simulink model "bacteriaPopulationStateflow"  (R2017b)
settings: Solver=FixedStepDiscrete  StartTime=0.0  StopTime=10.0  FixedStep=1  RelTol=1e-3
model workspace (MAT data in the model file):
  ContractValidatorBlocksMap = containers.Map
  ContractValidatorBlocksMap.serialization.keys = {'bacteriaPopulationStateflow/bacteriaPopulationSpec/validator', 'bacteriaPopulationStateflow1/bacteriaPopulationSpec/validator'}
  ContractValidatorBlocksMap.serialization.values{1}.block = 'bacteriaPopulationStateflow/bacteriaPopulationSpec/validator'
  ContractValidatorBlocksMap.serialization.values{1}.assumePorts = 1
  ContractValidatorBlocksMap.serialization.values{1}.guaranteePorts = 4
  ContractValidatorBlocksMap.serialization.values{1}.modeBlocksPorts = 3
  ContractValidatorBlocksMap.serialization.values{1}.portHandles.Inport = [309.000366211 310.00012207 311.00012207 312.00012207 313.00012207 314.00012207 315.00012207 316.00012207]
  ContractValidatorBlocksMap.serialization.values{1}.portHandles.Outport = 317.00012207
  ContractValidatorBlocksMap.serialization.values{1}.portHandles.Enable = []
  ContractValidatorBlocksMap.serialization.values{1}.portHandles.Trigger = []
  ContractValidatorBlocksMap.serialization.values{1}.portHandles.State = []
  ContractValidatorBlocksMap.serialization.values{1}.portHandles.LConn = []
  ContractValidatorBlocksMap.serialization.values{1}.portHandles.RConn = []
  ContractValidatorBlocksMap.serialization.values{1}.portHandles.Ifaction = []
  ContractValidatorBlocksMap.serialization.values{1}.portHandles.Reset = []
  ContractValidatorBlocksMap.serialization.values{1}.portConnectivity(1).Type = '1'
  ContractValidatorBlocksMap.serialization.values{1}.portConnectivity(1).Position = [360 -280]
  ContractValidatorBlocksMap.serialization.values{1}.portConnectivity(1).SrcBlock = 21.0001220703
  ContractValidatorBlocksMap.serialization.values{1}.portConnectivity(1).SrcPort = 0
  ContractValidatorBlocksMap.serialization.values{1}.portConnectivity(1).DstBlock = []
  ContractValidatorBlocksMap.serialization.values{1}.portConnectivity(1).DstPort = []
  ContractValidatorBlocksMap.serialization.values{1}.portConnectivity(2).Type = '2'
  ContractValidatorBlocksMap.serialization.values{1}.portConnectivity(2).Position = [360 -170]
  ContractValidatorBlocksMap.serialization.values{1}.portConnectivity(2).SrcBlock = 81.0001220703
  ContractValidatorBlocksMap.serialization.values{1}.portConnectivity(2).SrcPort = 0
  ContractValidatorBlocksMap.serialization.values{1}.portConnectivity(2).DstBlock = []
  ContractValidatorBlocksMap.serialization.values{1}.portConnectivity(2).DstPort = []
  ContractValidatorBlocksMap.serialization.values{1}.portConnectivity(3).Type = '3'
  ContractValidatorBlocksMap.serialization.values{1}.portConnectivity(3).Position = [360 -60]
  ContractValidatorBlocksMap.serialization.values{1}.portConnectivity(3).SrcBlock = 87.0003662109
  ContractValidatorBlocksMap.serialization.values{1}.portConnectivity(3).SrcPort = 0
  ContractValidatorBlocksMap.serialization.values{1}.portConnectivity(3).DstBlock = []
  ContractValidatorBlocksMap.serialization.values{1}.portConnectivity(3).DstPort = []
  ContractValidatorBlocksMap.serialization.values{1}.portConnectivity(4).Type = '4'
  ContractValidatorBlocksMap.serialization.values{1}.portConnectivity(4).Position = [360 50]
  ContractValidatorBlocksMap.serialization.values{1}.portConnectivity(4).SrcBlock = 99.0003662109
  ContractValidatorBlocksMap.serialization.values{1}.portConnectivity(4).SrcPort = 0
  ContractValidatorBlocksMap.serialization.values{1}.portConnectivity(4).DstBlock = []
  ContractValidatorBlocksMap.serialization.values{1}.portConnectivity(4).DstPort = []
  ContractValidatorBlocksMap.serialization.values{1}.portConnectivity(5).Type = '5'
  ContractValidatorBlocksMap.serialization.values{1}.portConnectivity(5).Position = [360 160]
  ContractValidatorBlocksMap.serialization.values{1}.portConnectivity(5).SrcBlock = 148.000366211
  ContractValidatorBlocksMap.serialization.values{1}.portConnectivity(5).SrcPort = 0
  ContractValidatorBlocksMap.serialization.values{1}.portConnectivity(5).DstBlock = []
  ContractValidatorBlocksMap.serialization.values{1}.portConnectivity(5).DstPort = []
  ContractValidatorBlocksMap.serialization.values{1}.portConnectivity(6).Type = '6'
  ContractValidatorBlocksMap.serialization.values{1}.portConnectivity(6).Position = [360 270]
  ContractValidatorBlocksMap.serialization.values{1}.portConnectivity(6).SrcBlock = 197.000366211
  ContractValidatorBlocksMap.serialization.values{1}.portConnectivity(6).SrcPort = 0
  ContractValidatorBlocksMap.serialization.values{1}.portConnectivity(6).DstBlock = []
  ContractValidatorBlocksMap.serialization.values{1}.portConnectivity(6).DstPort = []
  ContractValidatorBlocksMap.serialization.values{1}.portConnectivity(7).Type = '7'
  ContractValidatorBlocksMap.serialization.values{1}.portConnectivity(7).Position = [360 380]
  ContractValidatorBlocksMap.serialization.values{1}.portConnectivity(7).SrcBlock = 27.0003662109
  ContractValidatorBlocksMap.serialization.values{1}.portConnectivity(7).SrcPort = 0
  ContractValidatorBlocksMap.serialization.values{1}.portConnectivity(7).DstBlock = []
  ContractValidatorBlocksMap.serialization.values{1}.portConnectivity(7).DstPort = []
  ContractValidatorBlocksMap.serialization.values{1}.portConnectivity(8).Type = '8'
  ContractValidatorBlocksMap.serialization.values{1}.portConnectivity(8).Position = [360 490]
  ContractValidatorBlocksMap.serialization.values{1}.portConnectivity(8).SrcBlock = 238.000366211
  ContractValidatorBlocksMap.serialization.values{1}.portConnectivity(8).SrcPort = 0
  ContractValidatorBlocksMap.serialization.values{1}.portConnectivity(8).DstBlock = []
  ContractValidatorBlocksMap.serialization.values{1}.portConnectivity(8).DstPort = []
  ContractValidatorBlocksMap.serialization.values{1}.portConnectivity(9).Type = '1'
  ContractValidatorBlocksMap.serialization.values{1}.portConnectivity(9).Position = [500 105]
  ContractValidatorBlocksMap.serialization.values{1}.portConnectivity(9).SrcBlock = []
  ContractValidatorBlocksMap.serialization.values{1}.portConnectivity(9).SrcPort = []
  ContractValidatorBlocksMap.serialization.values{1}.portConnectivity(9).DstBlock = [250.00012207 20.0001220703]
  ContractValidatorBlocksMap.serialization.values{1}.portConnectivity(9).DstPort = [0 0]
  ContractValidatorBlocksMap.serialization.values{2}.block = 'bacteriaPopulationStateflow1/bacteriaPopulationSpec/validator'
  ContractValidatorBlocksMap.serialization.values{2}.assumePorts = 1
  ContractValidatorBlocksMap.serialization.values{2}.guaranteePorts = 4
  ContractValidatorBlocksMap.serialization.values{2}.modeBlocksPorts = 3
  ContractValidatorBlocksMap.serialization.values{2}.portHandles.Inport = [309.001586914 310.001220703 311.000854492 312.000976562 313.000976562 314.001098633 315.000976562 316.000854492]
  ContractValidatorBlocksMap.serialization.values{2}.portHandles.Outport = 317.001098633
  ContractValidatorBlocksMap.serialization.values{2}.portHandles.Enable = []
  ContractValidatorBlocksMap.serialization.values{2}.portHandles.Trigger = []
  ContractValidatorBlocksMap.serialization.values{2}.portHandles.State = []
  ContractValidatorBlocksMap.serialization.values{2}.portHandles.LConn = []
  ContractValidatorBlocksMap.serialization.values{2}.portHandles.RConn = []
  ContractValidatorBlocksMap.serialization.values{2}.portHandles.Ifaction = []
  ContractValidatorBlocksMap.serialization.values{2}.portHandles.Reset = []
  ContractValidatorBlocksMap.serialization.values{2}.portConnectivity(1).Type = '1'
  ContractValidatorBlocksMap.serialization.values{2}.portConnectivity(1).Position = [360 -280]
  ContractValidatorBlocksMap.serialization.values{2}.portConnectivity(1).SrcBlock = 21.0007324219
  ContractValidatorBlocksMap.serialization.values{2}.portConnectivity(1).SrcPort = 0
  ContractValidatorBlocksMap.serialization.values{2}.portConnectivity(1).DstBlock = []
  ContractValidatorBlocksMap.serialization.values{2}.portConnectivity(1).DstPort = []
  ContractValidatorBlocksMap.serialization.values{2}.portConnectivity(2).Type = '2'
  ContractValidatorBlocksMap.serialization.values{2}.portConnectivity(2).Position = [360 -170]
  ContractValidatorBlocksMap.serialization.values{2}.portConnectivity(2).SrcBlock = 81.0010986328
  ContractValidatorBlocksMap.serialization.values{2}.portConnectivity(2).SrcPort = 0
  ContractValidatorBlocksMap.serialization.values{2}.portConnectivity(2).DstBlock = []
  ContractValidatorBlocksMap.serialization.values{2}.portConnectivity(2).DstPort = []
  ContractValidatorBlocksMap.serialization.values{2}.portConnectivity(3).Type = '3'
  ContractValidatorBlocksMap.serialization.values{2}.portConnectivity(3).Position = [360 -60]
  ContractValidatorBlocksMap.serialization.values{2}.portConnectivity(3).SrcBlock = 87.0009765625
  ContractValidatorBlocksMap.serialization.values{2}.portConnectivity(3).SrcPort = 0
  ContractValidatorBlocksMap.serialization.values{2}.portConnectivity(3).DstBlock = []
  ContractValidatorBlocksMap.serialization.values{2}.portConnectivity(3).DstPort = []
  ContractValidatorBlocksMap.serialization.values{2}.portConnectivity(4).Type = '4'
  ContractValidatorBlocksMap.serialization.values{2}.portConnectivity(4).Position = [360 50]
  ContractValidatorBlocksMap.serialization.values{2}.portConnectivity(4).SrcBlock = 99.0009765625
  ContractValidatorBlocksMap.serialization.values{2}.portConnectivity(4).SrcPort = 0
  ContractValidatorBlocksMap.serialization.values{2}.portConnectivity(4).DstBlock = []
  ContractValidatorBlocksMap.serialization.values{2}.portConnectivity(4).DstPort = []
  ContractValidatorBlocksMap.serialization.values{2}.portConnectivity(5).Type = '5'
  ContractValidatorBlocksMap.serialization.values{2}.portConnectivity(5).Position = [360 160]
  ContractValidatorBlocksMap.serialization.values{2}.portConnectivity(5).SrcBlock = 148.000976562
  ContractValidatorBlocksMap.serialization.values{2}.portConnectivity(5).SrcPort = 0
  ContractValidatorBlocksMap.serialization.values{2}.portConnectivity(5).DstBlock = []
  ContractValidatorBlocksMap.serialization.values{2}.portConnectivity(5).DstPort = []
  ContractValidatorBlocksMap.serialization.values{2}.portConnectivity(6).Type = '6'
  ContractValidatorBlocksMap.serialization.values{2}.portConnectivity(6).Position = [360 270]
  ContractValidatorBlocksMap.serialization.values{2}.portConnectivity(6).SrcBlock = 197.000976562
  ContractValidatorBlocksMap.serialization.values{2}.portConnectivity(6).SrcPort = 0
  ContractValidatorBlocksMap.serialization.values{2}.portConnectivity(6).DstBlock = []
  ContractValidatorBlocksMap.serialization.values{2}.portConnectivity(6).DstPort = []
  ContractValidatorBlocksMap.serialization.values{2}.portConnectivity(7).Type = '7'
  ContractValidatorBlocksMap.serialization.values{2}.portConnectivity(7).Position = [360 380]
  ContractValidatorBlocksMap.serialization.values{2}.portConnectivity(7).SrcBlock = 27.0018310547
  ContractValidatorBlocksMap.serialization.values{2}.portConnectivity(7).SrcPort = 0
  ContractValidatorBlocksMap.serialization.values{2}.portConnectivity(7).DstBlock = []
  ContractValidatorBlocksMap.serialization.values{2}.portConnectivity(7).DstPort = []
  ContractValidatorBlocksMap.serialization.values{2}.portConnectivity(8).Type = '8'
  ContractValidatorBlocksMap.serialization.values{2}.portConnectivity(8).Position = [360 490]
  ContractValidatorBlocksMap.serialization.values{2}.portConnectivity(8).SrcBlock = 238.000976562
  ContractValidatorBlocksMap.serialization.values{2}.portConnectivity(8).SrcPort = 0
  ContractValidatorBlocksMap.serialization.values{2}.portConnectivity(8).DstBlock = []
  ContractValidatorBlocksMap.serialization.values{2}.portConnectivity(8).DstPort = []
  ContractValidatorBlocksMap.serialization.values{2}.portConnectivity(9).Type = '1'
  ContractValidatorBlocksMap.serialization.values{2}.portConnectivity(9).Position = [500 105]
  ContractValidatorBlocksMap.serialization.values{2}.portConnectivity(9).SrcBlock = []
  ContractValidatorBlocksMap.serialization.values{2}.portConnectivity(9).SrcPort = []
  ContractValidatorBlocksMap.serialization.values{2}.portConnectivity(9).DstBlock = [250.000488281 20.0009765625]
  ContractValidatorBlocksMap.serialization.values{2}.portConnectivity(9).DstPort = [0 0]
  ContractValidatorBlocksMap.serialization.uniformity = 0
  ContractValidatorBlocksMap.serialization.keyType = 'char'
  ContractValidatorBlocksMap.serialization.valueType = 'any'
undefined symbols (not defined in the file or in its folder): contractAfterSimulation, ContractAssumeBlock, contractBeforeSimulation, ContractBlock, ContractEnsureBlock, ContractGuaranteeBlock, ContractModeBlock, ContractRequireBlock, ContractValidatorBlock, saveValidatorParameters
libraries: Kind x14, simulink x2
settings Model: Creator=Mudathir  LastModifiedBy=mudat
settings CodeAppCC: StateflowObjectComments=on

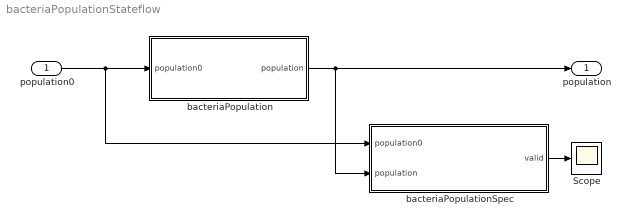
== system bacteriaPopulationStateflow ==
  population0 : Inport
  Scope : Scope
  bacteriaPopulation : Stateflow chart  TreatAsAtomicUnit=on
  bacteriaPopulationSpec : Subsystem  mask{ContractBlockType=ContractBlock}
      mask init:
      | set_param(gcb, 'LinkStatus', 'none');
      mask DialogControl DescTextVar Prompt: Contract block
      mask Display:
      | text(0.5, 0.5, '{\bf\fontsize{20}Contract}', 'hor', 'center', 'texmode','on');
      | blocks = find_system(gcb, 'LookUnderMasks','all', 'SearchDepth',1,'BlockType','Inport');
      | for i = 1 : length(blocks)
      |     blockName = get_param(blocks(i), 'Name');
      |     [path, blockName] = fileparts(char(blockName));
      |     port_label('input', i, blockName);
      | end
      | 
      | blocks = find_system(gcb, 'LookUnderMasks','all', 'SearchDepth',1,'BlockType','Outport');
      | for i = 1 : length(blocks)
      |     blockName = get_param(blocks(i), 'Name');
      |     [path, blockName] = fileparts(char(blockName));
      |     port_label('output', i, blockName);
      | end
  population : Outport
  wires:
  population0/1 -> bacteriaPopulation/1(population0), bacteriaPopulationSpec/1(population0)
  bacteriaPopulation/1(population) -> bacteriaPopulationSpec/2(population), population/1
  bacteriaPopulationSpec/1(valid) -> Scope/1

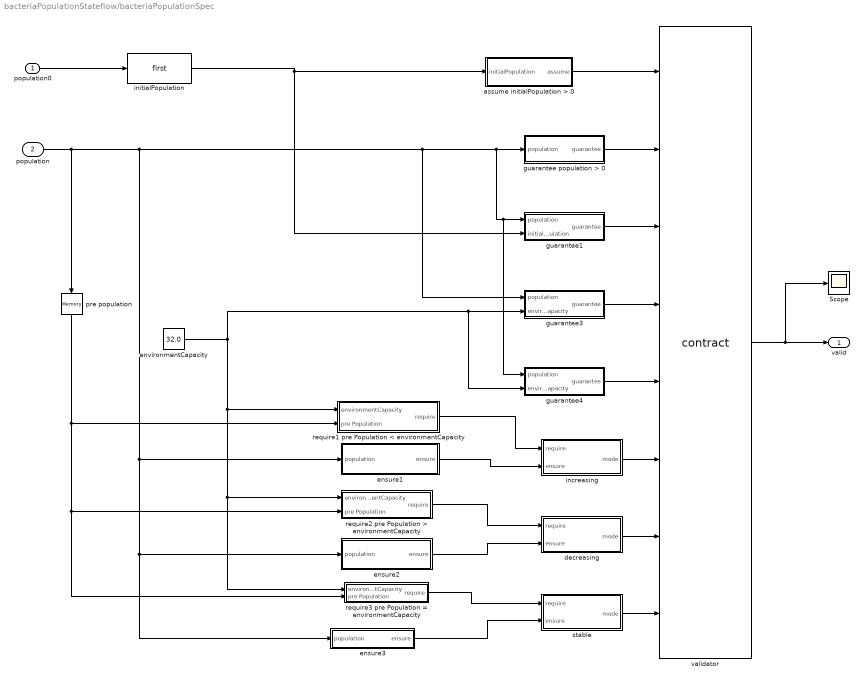
== system bacteriaPopulationStateflow/bacteriaPopulationSpec ==
  population0 : Inport
  population : Inport  Port=2
  Scope : Scope
  assume initialPopulation > 0 : Subsystem  mask{ContractBlockType=ContractAssumeBlock}
      mask init:
      | set_param(gcb, 'LinkStatus', 'none');
      mask DialogControl DescTextVar Prompt: Assume block
  decreasing : Subsystem  mask{ContractBlockType=ContractModeBlock}
      mask init:
      | set_param(gcb, 'LinkStatus', 'none');
      mask DialogControl DescTextVar Prompt: Mode block
  ensure1 : Subsystem  mask{ContractBlockType=ContractEnsureBlock}
      mask init:
      | set_param(gcb, 'LinkStatus', 'none');
      mask DialogControl DescTextVar Prompt: Ensure block
  ensure2 : Subsystem  mask{ContractBlockType=ContractEnsureBlock}
      mask init:
      | set_param(gcb, 'LinkStatus', 'none');
      mask DialogControl DescTextVar Prompt: Ensure block
  ensure3 : Subsystem  mask{ContractBlockType=ContractEnsureBlock}
      mask init:
      | set_param(gcb, 'LinkStatus', 'none');
      mask DialogControl DescTextVar Prompt: Ensure block
  environmentCapacity : Constant  Value=32.0  OutDataTypeStr=double
  guarantee population > 0 : Subsystem  mask{ContractBlockType=ContractGuaranteeBlock}
      mask init:
      | set_param(gcb, 'LinkStatus', 'none');
      mask DialogControl DescTextVar Prompt: Guarantee block
  guarantee1 : Subsystem  mask{ContractBlockType=ContractGuaranteeBlock}
      mask init:
      | set_param(gcb, 'LinkStatus', 'none');
      mask DialogControl DescTextVar Prompt: Guarantee block
  guarantee3 : Subsystem  mask{ContractBlockType=ContractGuaranteeBlock}
      mask init:
      | set_param(gcb, 'LinkStatus', 'none');
      mask DialogControl DescTextVar Prompt: Guarantee block
  guarantee4 : Subsystem  mask{ContractBlockType=ContractGuaranteeBlock}
      mask init:
      | set_param(gcb, 'LinkStatus', 'none');
      mask DialogControl DescTextVar Prompt: Guarantee block
  increasing : Subsystem  mask{ContractBlockType=ContractModeBlock}
      mask init:
      | set_param(gcb, 'LinkStatus', 'none');
      mask DialogControl DescTextVar Prompt: Mode block
  initialPopulation : Kind/first  SystemSampleTime=-1
      settings: SourceProductName=Kind lib
  pre population : Memory
  require1 pre Population < environmentCapacity : Subsystem  mask{ContractBlockType=ContractRequireBlock}
      mask init:
      | set_param(gcb, 'LinkStatus', 'none');
      mask DialogControl DescTextVar Prompt: Require block
  require2 pre Population > environmentCapacity : Subsystem  mask{ContractBlockType=ContractRequireBlock}
      mask init:
      | set_param(gcb, 'LinkStatus', 'none');
      mask DialogControl DescTextVar Prompt: Require block
  require3 pre Population = environmentCapacity : Subsystem  mask{ContractBlockType=ContractRequireBlock}
      mask init:
      | set_param(gcb, 'LinkStatus', 'none');
      mask DialogControl DescTextVar Prompt: Require block
  stable : Subsystem  mask{ContractBlockType=ContractModeBlock}
      mask init:
      | set_param(gcb, 'LinkStatus', 'none');
      mask DialogControl DescTextVar Prompt: Mode block
  validator : M-S-Function  LoadFcn=saveValidatorParameters(gcb);  InitFcn=contractBeforeSimulation();  StopFcn=contractAfterSimulation();  FunctionName=contract  mask(KindContractValidator){assumePorts=1, guaranteePorts=4, modePorts=3, ContractBlockType=ContractValidatorBlock, createInportsCheckbox=off, createEnsureRequireCheckbox=off}
      mask prompts: assumePorts "Assume ports     :"; guaranteePorts "Guarantee ports :"; modePorts "Mode ports        :"; createInportsCheckbox "Create inports and connect them automatically"; createEnsureRequireCheckbox "Create ensure and require blocks for mode blocks"
      mask init:
      | set_param(gcb,'LinkStatus','none');
      | contract_callback('inputs_callback',gcb);
      mask DialogControl DescTextVar Prompt: The validator block implements the following logic: <br> <br> <b>Sofar</b>(assume<sub>1</sub> <b>&#8743;</b> assume<sub>2</sub> <b>&#8743;</b> ... assume<sub>k</sub>) <b>&rarr;</b> (guarantee<sub>1</sub> <b>&#8743;</b> guarantee<sub>2</sub> <b>&#8743;</b> ... guarantee<sub>m</sub> <b>&#8743;</b>  mode<sub>1</sub> <b>&#8743;</b> mode<sub>2</sub> <b>&#8743;</b> ... <b>&#8743;</b> mode<sub>n</sub> )<br> where mode<sub>i</sub> = require<sub>i</sub> <b>&rarr;</b> ensure<sub>i</sub>
      mask Display:
      | color('black');
      | port_label('input',1,'assume');
      | port_label('input',2,'guarantee');
      | port_label('input',3,'guarantee');
      | port_label('input',4,'guarantee');
      | port_label('input',5,'guarantee');
      | port_label('input',6,'mode');
      | port_label('input',7,'mode');
      | port_label('input',8,'mode');
      | port_label('output',1,'valid');
  valid : Outport
  wires:
  validator/1 -> Scope/1, valid/1
  population0/1 -> initialPopulation/1
  population/1 -> pre population/1, ensure1/1(population), ensure3/1(population), ensure2/1(population), guarantee4/1(population), guarantee1/1(population), guarantee population > 0/1(population), guarantee3/1(population)
  require1 pre Population < environmentCapacity/1(require) -> increasing/1(require)
  ensure1/1(ensure) -> increasing/2(ensure)
  require2 pre Population > environmentCapacity/1(require) -> decreasing/1(require)
  ensure2/1(ensure) -> decreasing/2(ensure)
  require3 pre Population = environmentCapacity/1(require) -> stable/1(require)
  ensure3/1(ensure) -> stable/2(ensure)
  environmentCapacity/1 -> require3 pre Population = environmentCapacity/1(environmentCapacity), require2 pre Population > environmentCapacity/1(environmentCapacity), require1 pre Population < environmentCapacity/1(environmentCapacity), guarantee4/2(environmentCapacity), guarantee3/2(environmentCapacity)
  initialPopulation/1 -> assume initialPopulation > 0/1(initialPopulation), guarantee1/2(initialPopulation)
  assume initialPopulation > 0/1(assume) -> validator/1
  guarantee population > 0/1(guarantee) -> validator/2
  guarantee1/1(guarantee) -> validator/3
  guarantee3/1(guarantee) -> validator/4
  increasing/1(mode) -> validator/6
  decreasing/1(mode) -> validator/7
  stable/1(mode) -> validator/8
  guarantee4/1(guarantee) -> validator/5
  pre population/1 -> require1 pre Population < environmentCapacity/2(pre Population), require2 pre Population > environmentCapacity/2(pre Population), require3 pre Population = environmentCapacity/2(pre Population)

== system bacteriaPopulationStateflow/bacteriaPopulationSpec/assume initialPopulation > 0 ==
  initialPopulation : Inport
  Compare To Zero : simulink/Logic and Bit Operations/Compare To Zero  relop=>  OutDataTypeStr=boolean
  assume : Outport  OutDataTypeStr=boolean
  wires:
  initialPopulation/1 -> Compare To Zero/1
  Compare To Zero/1 -> assume/1

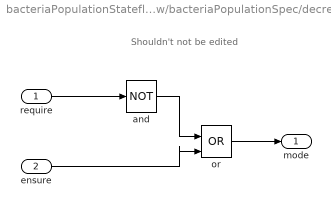
== system bacteriaPopulationStateflow/bacteriaPopulationSpec/decreasing ==
  note: Shouldn't not be edited
  require : Inport  OutDataTypeStr=boolean
  ensure : Inport  Port=2  OutDataTypeStr=boolean
  and : Logic  Operator=NOT  IconShape=distinctive  AllPortsSameDT=off  OutDataTypeStr=boolean
  or : Logic  Operator=OR  IconShape=distinctive  AllPortsSameDT=off  OutDataTypeStr=boolean
  mode : Outport
  wires:
  require/1 -> and/1
  ensure/1 -> or/2
  and/1 -> or/1
  or/1 -> mode/1

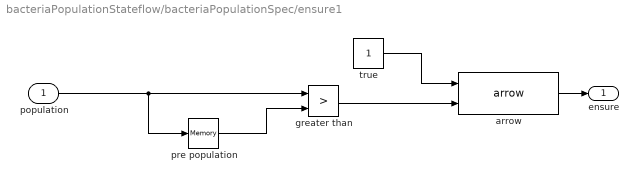
== system bacteriaPopulationStateflow/bacteriaPopulationSpec/ensure1 ==
  population : Inport
  arrow : Kind/arrow  LustreOperatorBlock=ArrowOperator
      settings: SourceProductName=Kind lib
  greater than : RelationalOperator  Operator=>  OutDataTypeStr=boolean  RndMeth=Simplest
  pre population : Memory
  true : Constant  OutDataTypeStr=boolean
  ensure : Outport  OutDataTypeStr=boolean
  wires:
  pre population/1 -> greater than/2
  true/1 -> arrow/1
  greater than/1 -> arrow/2
  arrow/1 -> ensure/1
  population/1 -> pre population/1, greater than/1

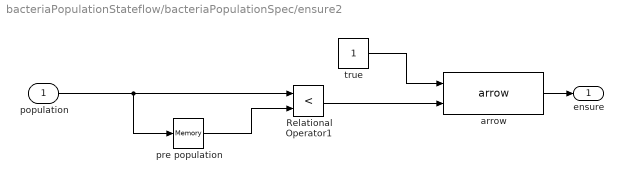
== system bacteriaPopulationStateflow/bacteriaPopulationSpec/ensure2 ==
  population : Inport
  Relational Operator1 : RelationalOperator  Operator=<  OutDataTypeStr=boolean  RndMeth=Simplest
  arrow : Kind/arrow  LustreOperatorBlock=ArrowOperator
      settings: SourceProductName=Kind lib
  pre population : Memory
  true : Constant  OutDataTypeStr=boolean
  ensure : Outport  OutDataTypeStr=boolean
  wires:
  pre population/1 -> Relational Operator1/2
  true/1 -> arrow/1
  Relational Operator1/1 -> arrow/2
  arrow/1 -> ensure/1
  population/1 -> pre population/1, Relational Operator1/1

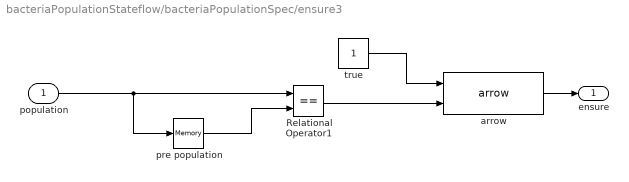
== system bacteriaPopulationStateflow/bacteriaPopulationSpec/ensure3 ==
  population : Inport
  Relational Operator1 : RelationalOperator  Operator===  OutDataTypeStr=boolean  RndMeth=Simplest
  arrow : Kind/arrow  LustreOperatorBlock=ArrowOperator
      settings: SourceProductName=Kind lib
  pre population : Memory
  true : Constant  OutDataTypeStr=boolean
  ensure : Outport  OutDataTypeStr=boolean
  wires:
  Relational Operator1/1 -> arrow/2
  true/1 -> arrow/1
  arrow/1 -> ensure/1
  population/1 -> pre population/1, Relational Operator1/1
  pre population/1 -> Relational Operator1/2

== system bacteriaPopulationStateflow/bacteriaPopulationSpec/guarantee population > 0 ==
  population : Inport
  Compare To Zero1 : simulink/Logic and Bit Operations/Compare To Zero  relop=>  OutDataTypeStr=boolean
  guarantee : Outport  OutDataTypeStr=boolean
  wires:
  population/1 -> Compare To Zero1/1
  Compare To Zero1/1 -> guarantee/1

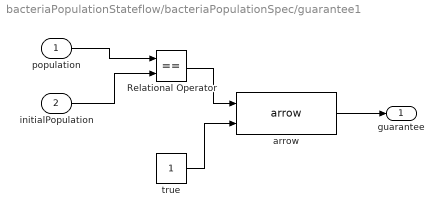
== system bacteriaPopulationStateflow/bacteriaPopulationSpec/guarantee1 ==
  population : Inport
  initialPopulation : Inport  Port=2
  Relational Operator : RelationalOperator  Operator===  OutDataTypeStr=boolean  RndMeth=Simplest
  arrow : Kind/arrow  LustreOperatorBlock=ArrowOperator
      settings: SourceProductName=Kind lib
  true : Constant  OutDataTypeStr=boolean
  guarantee : Outport  OutDataTypeStr=boolean
  wires:
  arrow/1 -> guarantee/1
  true/1 -> arrow/2
  population/1 -> Relational Operator/1
  initialPopulation/1 -> Relational Operator/2
  Relational Operator/1 -> arrow/1

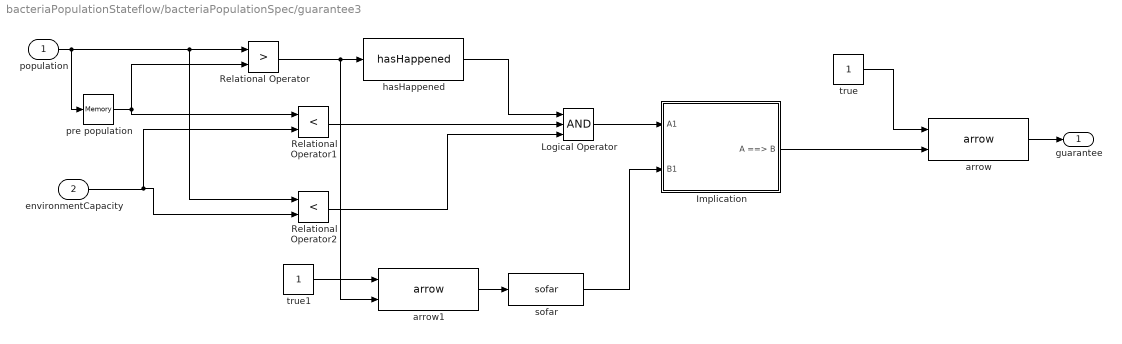
== system bacteriaPopulationStateflow/bacteriaPopulationSpec/guarantee3 ==
  population : Inport
  environmentCapacity : Inport  Port=2
  Implication : Subsystem  mask(CoCoSim-Implies){}
      mask help: CoCoSim block for Logical Implication
      mask Display: disp(' ')
  Logical Operator : Logic  Inputs=3  AllPortsSameDT=off  OutDataTypeStr=boolean
  Relational Operator : RelationalOperator  Operator=>  OutDataTypeStr=boolean  RndMeth=Simplest
  Relational Operator1 : RelationalOperator  Operator=<  OutDataTypeStr=boolean  RndMeth=Simplest
  Relational Operator2 : RelationalOperator  Operator=<  OutDataTypeStr=boolean  RndMeth=Simplest
  arrow : Kind/arrow  LustreOperatorBlock=ArrowOperator
      settings: SourceProductName=Kind lib
  arrow1 : Kind/arrow  LustreOperatorBlock=ArrowOperator
      settings: SourceProductName=Kind lib
  hasHappened : Kind/hasHappened  SystemSampleTime=-1
      settings: SourceProductName=Kind lib
  pre population : Memory
  sofar : Kind/sofar  SystemSampleTime=-1
      settings: SourceProductName=Kind lib
  true : Constant  OutDataTypeStr=boolean
  true1 : Constant  OutDataTypeStr=boolean
  guarantee : Outport  OutDataTypeStr=boolean
  wires:
  population/1 -> pre population/1, Relational Operator2/1, Relational Operator/1
  pre population/1 -> Relational Operator1/1, Relational Operator/2
  Relational Operator/1 -> arrow1/2, hasHappened/1
  hasHappened/1 -> Logical Operator/1
  environmentCapacity/1 -> Relational Operator2/2, Relational Operator1/2
  arrow/1 -> guarantee/1
  Relational Operator1/1 -> Logical Operator/2
  Relational Operator2/1 -> Logical Operator/3
  true/1 -> arrow/1
  true1/1 -> arrow1/1
  Logical Operator/1 -> Implication/1(A1)
  sofar/1 -> Implication/2(B1)
  arrow1/1 -> sofar/1
  Implication/1(A ==> B) -> arrow/2

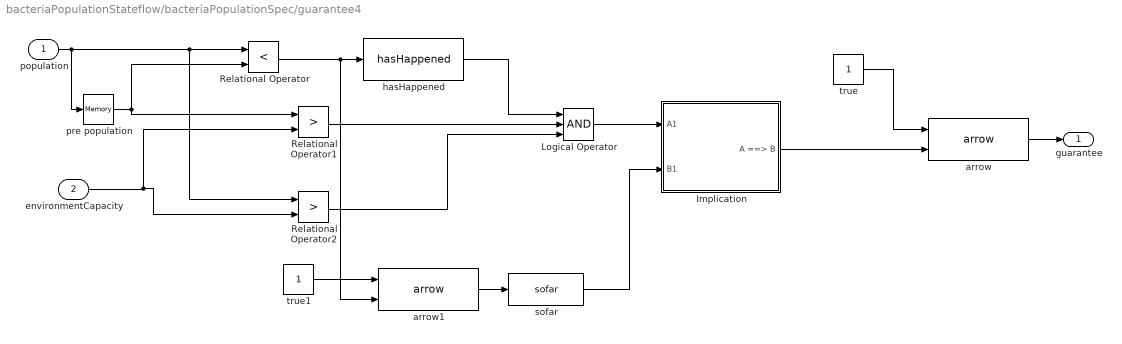
== system bacteriaPopulationStateflow/bacteriaPopulationSpec/guarantee4 ==
  population : Inport
  environmentCapacity : Inport  Port=2
  Implication : Subsystem  mask(CoCoSim-Implies){}
      mask help: CoCoSim block for Logical Implication
      mask Display: disp(' ')
  Logical Operator : Logic  Inputs=3  AllPortsSameDT=off  OutDataTypeStr=boolean
  Relational Operator : RelationalOperator  Operator=<  OutDataTypeStr=boolean  RndMeth=Simplest
  Relational Operator1 : RelationalOperator  Operator=>  OutDataTypeStr=boolean  RndMeth=Simplest
  Relational Operator2 : RelationalOperator  Operator=>  OutDataTypeStr=boolean  RndMeth=Simplest
  arrow : Kind/arrow  LustreOperatorBlock=ArrowOperator
      settings: SourceProductName=Kind lib
  arrow1 : Kind/arrow  LustreOperatorBlock=ArrowOperator
      settings: SourceProductName=Kind lib
  hasHappened : Kind/hasHappened  SystemSampleTime=-1
      settings: SourceProductName=Kind lib
  pre population : Memory
  sofar : Kind/sofar  SystemSampleTime=-1
      settings: SourceProductName=Kind lib
  true : Constant  OutDataTypeStr=boolean
  true1 : Constant  OutDataTypeStr=boolean
  guarantee : Outport  OutDataTypeStr=boolean
  wires:
  Relational Operator2/1 -> Logical Operator/3
  Implication/1(A ==> B) -> arrow/2
  true/1 -> arrow/1
  environmentCapacity/1 -> Relational Operator2/2, Relational Operator1/2
  sofar/1 -> Implication/2(B1)
  Relational Operator/1 -> arrow1/2, hasHappened/1
  arrow1/1 -> sofar/1
  population/1 -> pre population/1, Relational Operator2/1, Relational Operator/1
  pre population/1 -> Relational Operator1/1, Relational Operator/2
  arrow/1 -> guarantee/1
  Relational Operator1/1 -> Logical Operator/2
  Logical Operator/1 -> Implication/1(A1)
  true1/1 -> arrow1/1
  hasHappened/1 -> Logical Operator/1

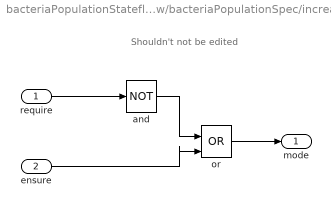
== system bacteriaPopulationStateflow/bacteriaPopulationSpec/increasing ==
  note: Shouldn't not be edited
  require : Inport  OutDataTypeStr=boolean
  ensure : Inport  Port=2  OutDataTypeStr=boolean
  and : Logic  Operator=NOT  IconShape=distinctive  AllPortsSameDT=off  OutDataTypeStr=boolean
  or : Logic  Operator=OR  IconShape=distinctive  AllPortsSameDT=off  OutDataTypeStr=boolean
  mode : Outport
  wires:
  require/1 -> and/1
  ensure/1 -> or/2
  and/1 -> or/1
  or/1 -> mode/1

== system bacteriaPopulationStateflow/bacteriaPopulationSpec/require1 pre Population < environmentCapacity ==
  environmentCapacity : Inport
  pre Population : Inport  Port=2
  Relational Operator : RelationalOperator  Operator=<  OutDataTypeStr=boolean  RndMeth=Simplest
  require : Outport  OutDataTypeStr=boolean
  wires:
  pre Population/1 -> Relational Operator/1
  environmentCapacity/1 -> Relational Operator/2
  Relational Operator/1 -> require/1

== system bacteriaPopulationStateflow/bacteriaPopulationSpec/require2 pre Population > environmentCapacity ==
  environmentCapacity : Inport
  pre Population : Inport  Port=2
  Relational Operator : RelationalOperator  Operator=>  OutDataTypeStr=boolean  RndMeth=Simplest
  require : Outport  OutDataTypeStr=boolean
  wires:
  pre Population/1 -> Relational Operator/1
  Relational Operator/1 -> require/1
  environmentCapacity/1 -> Relational Operator/2

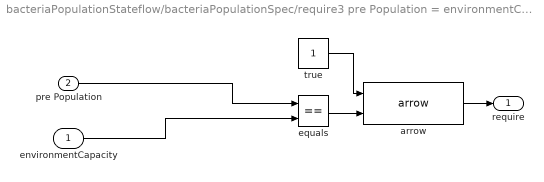
== system bacteriaPopulationStateflow/bacteriaPopulationSpec/require3 pre Population = environmentCapacity ==
  environmentCapacity : Inport
  pre Population : Inport  Port=2
  arrow : Kind/arrow  LustreOperatorBlock=ArrowOperator
      settings: SourceProductName=Kind lib
  equals : RelationalOperator  Operator===  OutDataTypeStr=boolean  RndMeth=Simplest
  true : Constant  OutDataTypeStr=boolean
  require : Outport  OutDataTypeStr=boolean
  wires:
  environmentCapacity/1 -> equals/2
  pre Population/1 -> equals/1
  true/1 -> arrow/1
  equals/1 -> arrow/2
  arrow/1 -> require/1

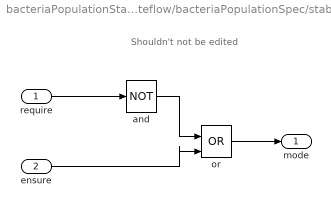
== system bacteriaPopulationStateflow/bacteriaPopulationSpec/stable ==
  note: Shouldn't not be edited
  require : Inport  OutDataTypeStr=boolean
  ensure : Inport  Port=2  OutDataTypeStr=boolean
  and : Logic  Operator=NOT  IconShape=distinctive  AllPortsSameDT=off  OutDataTypeStr=boolean
  or : Logic  Operator=OR  IconShape=distinctive  AllPortsSameDT=off  OutDataTypeStr=boolean
  mode : Outport
  wires:
  require/1 -> and/1
  ensure/1 -> or/2
  and/1 -> or/1
  or/1 -> mode/1

== system bacteriaPopulationStateflow/bacteriaPopulationSpec/guarantee3/Implication ==
  A1 : Inport
  B1 : Inport  Port=2
  Logical Operator : Logic  Operator=OR  AllPortsSameDT=off  OutDataTypeStr=boolean
  Logical Operator1 : Logic  Operator=NOT  AllPortsSameDT=off  OutDataTypeStr=boolean
  A ==> B : Outport
  wires:
  A1/1 -> Logical Operator1/1
  Logical Operator1/1 -> Logical Operator/1
  B1/1 -> Logical Operator/2
  Logical Operator/1 -> A ==> B/1

== system bacteriaPopulationStateflow/bacteriaPopulationSpec/guarantee4/Implication ==
  A1 : Inport
  B1 : Inport  Port=2
  Logical Operator : Logic  Operator=OR  AllPortsSameDT=off  OutDataTypeStr=boolean
  Logical Operator1 : Logic  Operator=NOT  AllPortsSameDT=off  OutDataTypeStr=boolean
  A ==> B : Outport
  wires:
  A1/1 -> Logical Operator1/1
  Logical Operator1/1 -> Logical Operator/1
  B1/1 -> Logical Operator/2
  Logical Operator/1 -> A ==> B/1

== stateflow chart bacteriaPopulationStateflow/bacteriaPopulation ==
  state increasing
    entry:
    prePopulation = population,
    population = prePopulation * 2.0;
    on dummyEvent: population = population;
    on after(5, dummyEvent): population = population;
    on before(5, dummyEvent): population = population;
    on at(5, dummyEvent): population = population;
    on every(5, dummyEvent): population = population;
  state stable
    entry:
    prePopulation = population;
  state start
    entry:
    prePopulation = population0;
    population = population0;
  state [x1,y1]=decrease(x,y) [function]
    (default) -> (junction 34) : {x1 = y; }
    (junction 34) -> (junction 38) : {y1 = x / 2.0;}
  state decreasing
    entry:
    [prePopulation,population] = ...
    decrease(prePopulation,  population);
  (default) -> start
  increasing -> (junction 13)
  (junction 13) -> increasing [order 1] : [population < 32.0]
  start -> (junction 13)
  (junction 13) -> stable [order 3] : [population == 32.0]
  (junction 13) -> decreasing [order 2] : [population > 32.0]
  decreasing -> (junction 13)
  data: x function_input; y function_input; x1 function_output; y1 function_output; population output; population0 input; prePopulation local
  events: dummyEvent local FUNCTION_CALL_EVENT
